simulink model "MPCNonModualNewTorque"  (R2015b)
settings: Solver=ode4  StartTime=0.0  StopTime=TMax  FixedStep=Ts  RelTol=1e-3
values from neighbouring files (symbols this model uses):
  DT = fscanf(fid,'    [YY_Read_FAST_Input.m]
  NDOF = 24    [YY_Read_FAST_Input.m]
  NumOuts = 2    [Reduced4to3_2DOF_18.mat]    (also in YY_Read_FAST_Input.m = 1)
  OutList = {}    [YY_Read_FAST_Input.m]
  q_init = zeros(1,NDOF)    [YY_Read_FAST_Input.m]
  qdot_init = zeros(1,NDOF)    [YY_Read_FAST_Input.m]
undefined symbols (not defined in the file or in its folder): strmatch
libraries: mpclib x1
settings Model: Creator=yuy13010  LastModifiedBy=yuy13010

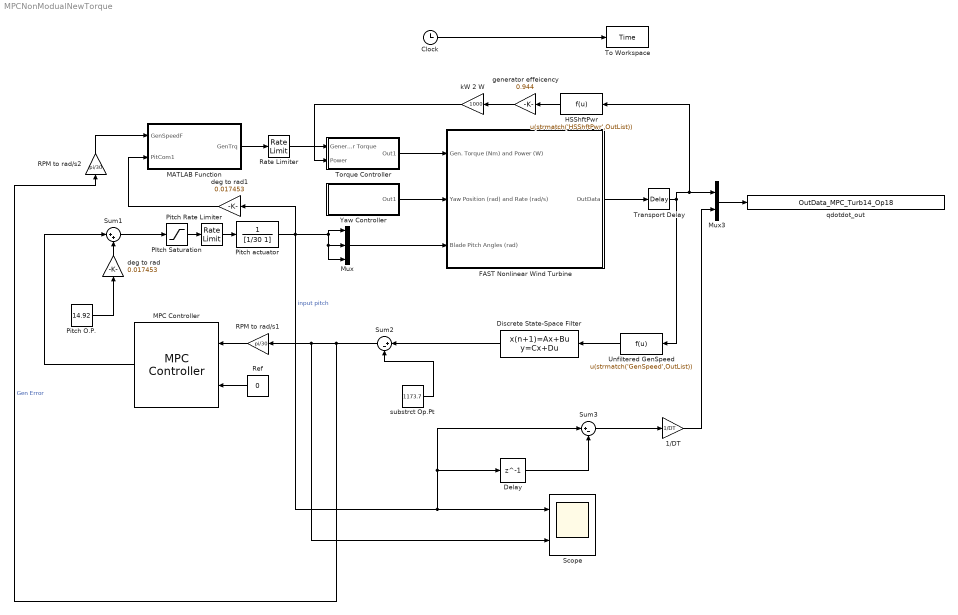
== system MPCNonModualNewTorque ==
  1/DT : Gain  Gain=1/DT  SaturateOnIntegerOverflow=on  OutDataTypeStr=Inherit: Same as input  ParamDataTypeStr=Inherit: Same as input
  Clock : Clock
  Delay : Delay  DelayLength=1
  Discrete State-Space Filter : DiscreteStateSpace  A=0.9806  B=0.0194  C=0.9806  D=0.0194  SampleTime=DT
  FAST Nonlinear Wind Turbine : Subsystem
  HSShftPwr : Fcn  Expr=u(strmatch('HSShftPwr',OutList))  SampleTime=DT
  MATLAB Function : MATLAB Function  TreatAsAtomicUnit=on
  MPC Controller : mpclib/MPC Controller  SCDEnableBlockLinearizationSpecification=on  mpcobj=mpcobj  x0=[]  is_multiple=0  enable_value=0  return_u0=off  ref_from_ws=off  ref_signal_name=[]  ref_preview=off  md_from_ws=off  md_signal_name=[]  md_preview=off  from_project=off  project_file=MPCtask.mat  md_inport=off  mv_inport=off  cost_outport=off  return_sequence=off  return_qpstatus=off  return_state=off  state_inport=off  lims_inport=off  ywt_inport=off  is_designfromscratch=0  uwt_inport=off  duwt_inport=off  rhoeps_inport=off  uref_inport=off  n_ts=0.0125  n_mv=1  n_md=0  n_ud=0  n_mo=1  n_uo=0  BlockDataType=double  SampleTimeInherited=off  switch_inport=off
  Mux : Mux  Inputs=3
  Mux3 : Mux  Inputs=2
  PItch Saturation : Saturate  UpperLimit=1.570796  LowerLimit=0  SampleTime=DT
  Pitch O.P. : Constant  Value=14.92
  Pitch Rate Limiter : RateLimiter  RisingSlewLimit=0.1396263  FallingSlewLimit=-0.1396263  SampleTimeMode=inherited
  Pitch actuator : TransferFcn  Denominator=[1/30 1]
  RPM to rad/s1 : Gain  Gain=pi/30  SaturateOnIntegerOverflow=on  OutDataTypeStr=Inherit: Same as input  ParamDataTypeStr=Inherit: Same as input
  RPM to rad/s2 : Gain  Gain=pi/30  SaturateOnIntegerOverflow=on  OutDataTypeStr=Inherit: Same as input  ParamDataTypeStr=Inherit: Same as input
  Rate Limiter : RateLimiter  RisingSlewLimit=15000  FallingSlewLimit=-15000  SampleTimeMode=inherited
  Ref : Constant  Value=0
  Scope : Scope  NumInputPorts=2
  Sum1 : Sum  Inputs=|++
  Sum2 : Sum  Inputs=|+-  SampleTime=DT
  Sum3 : Sum  Inputs=|+-  SampleTime=DT
  To Workspace : ToWorkspace  VariableName=Time  SampleTime=-1
  Torque Controller : Subsystem
  Transport Delay : TransportDelay  DelayTime=0.02
  Unfiltered GenSpeed : Fcn  Expr=u(strmatch('GenSpeed',OutList))  SampleTime=DT
  Yaw Controller : Subsystem
  deg to rad : Gain  Gain=0.017453  SaturateOnIntegerOverflow=on  OutDataTypeStr=Inherit: Same as input  ParamDataTypeStr=Inherit: Same as input
  deg to rad1 : Gain  Gain=0.017453  SaturateOnIntegerOverflow=on  OutDataTypeStr=Inherit: Same as input  ParamDataTypeStr=Inherit: Same as input
  generator effeicency : Gain  Gain=0.944  SaturateOnIntegerOverflow=on  OutDataTypeStr=Inherit: Same as input  ParamDataTypeStr=Inherit: Same as input
  kW 2 W : Gain  Gain=1000  SaturateOnIntegerOverflow=on  OutDataTypeStr=Inherit: Same as input  ParamDataTypeStr=Inherit: Same as input
  qdotdot_out : ToWorkspace  VariableName=OutData_MPC_Turb14_Op18  SampleTime=-1
  substrct Op.Pt : Constant  Value=1173.7
  wires:
  Clock/1 -> To Workspace/1
  Torque Controller/1(Out1) -> FAST Nonlinear Wind Turbine/1(Gen. Torque (Nm) and Power (W))
  Yaw Controller/1(Out1) -> FAST Nonlinear Wind Turbine/2(Yaw Position (rad) and Rate (rad/s))
  Mux/1 -> FAST Nonlinear Wind Turbine/3(Blade Pitch Angles (rad))
  substrct Op.Pt/1 -> Sum2/2
  Unfiltered GenSpeed/1 -> Discrete State-Space Filter/1
  Discrete State-Space Filter/1 -> Sum2/1
  FAST Nonlinear Wind Turbine/1(OutData) -> Transport Delay/1
  Pitch O.P./1 -> deg to rad/1
  deg to rad/1 -> Sum1/2
  Sum1/1 -> PItch Saturation/1
  PItch Saturation/1 -> Pitch Rate Limiter/1
  Pitch Rate Limiter/1 -> Pitch actuator/1
  MPC Controller/1 -> Sum1/1
  Ref/1 -> MPC Controller/2
  RPM to rad/s1/1 -> MPC Controller/1
  Pitch actuator/1 -> deg to rad1/1, Mux/1, Mux/3, Mux/2, Sum3/1, Delay/1, Scope/1  "input pitch"
  Delay/1 -> Sum3/2
  Sum3/1 -> 1/DT/1
  1/DT/1 -> Mux3/2
  Mux3/1 -> qdotdot_out/1
  Sum2/1 -> RPM to rad/s2/1, Scope/2, RPM to rad/s1/1  "Gen Error"
  MATLAB Function/1(GenTrq) -> Rate Limiter/1
  Rate Limiter/1 -> Torque Controller/1(Generator Torque)
  RPM to rad/s2/1 -> MATLAB Function/1(GenSpeedF)
  deg to rad1/1 -> MATLAB Function/2(PitCom1)
  Transport Delay/1 -> Unfiltered GenSpeed/1, Mux3/1, HSShftPwr/1
  HSShftPwr/1 -> generator effeicency/1
  generator effeicency/1 -> kW 2 W/1
  kW 2 W/1 -> Torque Controller/2(Power)

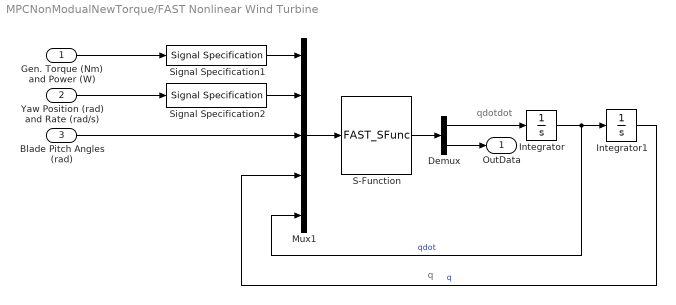
== system MPCNonModualNewTorque/FAST Nonlinear Wind Turbine ==
  note: qdotdot
  note: q
  Gen. Torque (Nm) and Power (W) : Inport
  Yaw Position (rad) and Rate (rad/s) : Inport  Port=2
  Blade Pitch Angles (rad) : Inport  Port=3
  Demux : Demux  Outputs=[NDOF, NumOuts]
  Integrator : Integrator  InitialCondition=qdot_init
  Integrator1 : Integrator  InitialCondition=q_init
  Mux1 : Mux  Inputs=5
  S-Function : S-Function  FunctionName=FAST_SFunc  SFunctionDeploymentMode=off  EnableBusSupport=off
  Signal Specification1 : SignalSpecification  OutDataTypeStr=double  Dimensions=2
  Signal Specification2 : SignalSpecification  OutDataTypeStr=double  Dimensions=2
  OutData : Outport
  wires:
  Integrator/1 -> Integrator1/1, Mux1/5  "qdot"
  Gen. Torque (Nm) and Power (W)/1 -> Signal Specification1/1
  S-Function/1 -> Demux/1
  Demux/1 -> Integrator/1
  Demux/2 -> OutData/1
  Mux1/1 -> S-Function/1
  Blade Pitch Angles (rad)/1 -> Mux1/3
  Yaw Position (rad) and Rate (rad/s)/1 -> Signal Specification2/1
  Integrator1/1 -> Mux1/4  "q"
  Signal Specification1/1 -> Mux1/1
  Signal Specification2/1 -> Mux1/2

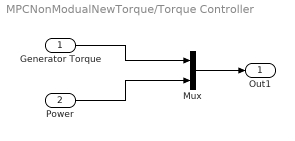
== system MPCNonModualNewTorque/Torque Controller ==
  Generator Torque : Inport
  Power : Inport  Port=2
  Mux : Mux  Inputs=2
  Out1 : Outport
  wires:
  Mux/1 -> Out1/1
  Generator Torque/1 -> Mux/1
  Power/1 -> Mux/2

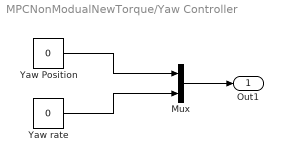
== system MPCNonModualNewTorque/Yaw Controller ==
  Mux : Mux  Inputs=2
  Yaw Position : Constant  Value=0
  Yaw rate : Constant  Value=0
  Out1 : Outport
  wires:
  Mux/1 -> Out1/1
  Yaw Position/1 -> Mux/1
  Yaw rate/1 -> Mux/2

== matlab function MPCNonModualNewTorque/MATLAB Function ==
  data: GenSpeedF input; GenTrq output; PitCom1 input
function GenTrq  = Torque(GenSpeedF,PitCom1)


%N.m                               rad/s    ,rad
%Torque controller
% PC_RefSpd = 122.9096;  % Desired (reference) HSS speed for pitch controller, rad/s.
% VS_MaxRat = 15000.0;  %Maximum torque rate (in absolute value) in torque controller, N-m/s.

VS_MaxTq  = 47402.91; %Maximum generator torque in Region 3 (HSS side), N-m. -- chosen to be 10% above VS_RtTq = 43.09355kNm
VS_Rgn2K  = 2.332287 ;%Generator torque constant in Region 2 (HSS side), N-m/(rad/s)^2.

VS_Rgn2Sp = 91.21091;  %Transitional generator speed (HSS side) between regions 1 1/2 and 2, rad/s.

VS_Rgn3MP = 0.01745329 ; %Minimum pitch angle at which the torque is computed as if we are in region 3 regardless of the generator speed, rad. -- chosen to be 1.0 degree above PC_MinPit

VS_RtGnSp = 121.6805;  %Rated generator speed (HSS side), rad/s. -- chosen to be 99% of PC_RefSpd
VS_RtPwr = 5296610.0;  %Rated generator generator power in Region 3, Watts. -- chosen to be 5MW divided by the electrical generator efficiency of 94.4%
VS_CtInSp  =   70.16224 ;   %Transitional generator speed (HSS side) between regions 1 and 1 1/2, rad/s.
VS_SlPc       =      10.0 ;                      %Rated generator slip percentage in Region 2 1/2, %.


% VS_Slope15      %Torque/speed slope of region 1 1/2 cut-in torque ramp , N-m/(rad/s).
% VS_Slope25      %Torque/speed slope of region 2 1/2 induction generator, N-m/(rad/s).
% VS_SySp         %Synchronous speed of region 2 1/2 induction generator, rad/s.
% VS_TrGnSp       %Transitional generator speed (HSS side) between regions 2 and 2 1/2, rad/s.


%Determine some torque control parameters not specified directly:

   VS_SySp    = VS_RtGnSp/( 1.0 +  0.01*VS_SlPc );
   VS_Slope15 = ( VS_Rgn2K*VS_Rgn2Sp*VS_Rgn2Sp )/( VS_Rgn2Sp - VS_CtInSp );
   VS_Slope25 = ( VS_RtPwr/VS_RtGnSp           )/( VS_RtGnSp - VS_SySp   );
   if ( VS_Rgn2K == 0.0 ) % .TRUE. if the Region 2 torque is flat, and thus, the denominator in the ELSE condition is zero
      VS_TrGnSp = VS_SySp;
   else                          % .TRUE. if the Region 2 torque is quadratic with speed
      VS_TrGnSp = ( VS_Slope25 - sqrt( VS_Slope25*( VS_Slope25 - 4.0*VS_Rgn2K*VS_SySp ) ) )/( 2.0*VS_Rgn2K );
   end
   
  % Variable-speed torque control:
 % Compute the generator torque, which depends on which region we are in:

      if ( (   GenSpeedF >= VS_RtGnSp ) || (  PitCom1 >= VS_Rgn3MP ) )    % We are in region 3 - power is constant
         GenTrq = VS_RtPwr/GenSpeedF;
      elseif ( GenSpeedF <= VS_CtInSp )                                   % We are in region 1 - torque is zero
         GenTrq = 0.0;
      elseif ( GenSpeedF <  VS_Rgn2Sp )                                    % We are in region 1 1/2 - linear ramp in torque from zero to optimal
         GenTrq = VS_Slope15*( GenSpeedF - VS_CtInSp );
      elseif ( GenSpeedF <  VS_TrGnSp )                                   % We are in region 2 - optimal torque is proportional to the square of the generator speed
         GenTrq = VS_Rgn2K*GenSpeedF*GenSpeedF;
      else                                                                %We are in region 2 1/2 - simple induction generator transition region
         GenTrq = VS_Slope25*( GenSpeedF - VS_SySp   );
      end
   %Saturate the commanded torque using the maximum torque limit:
   
   GenTrq = min (GenTrq, VS_MaxTq);   %Saturate the command using the maximum torque limit
   
   %Saturate the commanded torque using the torque rate limit:
   %use simulink block
